simulink model "grid_side_VOC_SteadyState3"  (R2013a)
settings: Solver=ode45  SolverMode=SingleTasking  StartTime=0.0  StopTime=30  FixedStep=0.00001  RelTol=1e-3
values from neighbouring files (symbols this model uses):
  Cdc = 1/(Omega_b*XCdc)    (= 0.0427146921878)    [grid_side_VOC_Constants.m]
  F0 = 1    [grid_side_VOC_Constants.m]
  Fb = 60    [grid_side_VOC_Constants.m]
  Fs = 2040    [grid_side_VOC_Constants.m]
  Fsampling = 10e3    (= 10000)    [grid_side_VOC_Constants.m]
  Grid_Angle_init = pi    (= 3.14159265359)    [grid_side_VOC_Constants.m]
  Ibase = (Pb/3)/(690/(3^0.5))    (= 1924.5008973)    [grid_side_VOC_Constants.m]
  iq_ref_pu = 0    [grid_side_VOC_Constants.m]
  Ki = 2    [grid_side_VOC_Constants.m]
  Kp = 1    [grid_side_VOC_Constants.m]
  Lgrid = 0.1098e-3    (= 0.0001098)    [grid_side_VOC_Constants.m]
  Rdc_series = 0.1*Zb    (= 0.0207)    [grid_side_VOC_Constants.m]
  Vbase = Vp/(2^.5)    (= 398.371685741)    [grid_side_VOC_Constants.m]
  Vdc_ref = 3.062    [grid_side_VOC_Constants.m]
  Vp = (690*(2^0.5))/(3^0.5)    (= 563.38264084)    [grid_side_VOC_Constants.m]
  XLgrid_pu = XLgrid/Zb    (= 0.2)    [grid_side_VOC_Constants.m]
libraries: powerlib x21, powerlib_extras x3, simulink x3, simulink_extras x2
settings Model: Creator=lang  LastModifiedBy=Sony
settings DataIOCC: SignalLoggingSaveFormat=ModelDataLogs
settings OptimizationCC: BlockReduction=off  BooleanDataType=off  InlineParams=on
settings DebuggingCC: SaveWithParameterizedLinksMsg=none  SignalResolutionControl=TryResolveAllWithWarning  SolverPrmCheckMsg=none  MultiTaskDSMMsg=warning  MultiTaskCondExecSysMsg=none  StrictBusMsg=None
settings HardwareCC: TargetUnknown=on
settings RTWCC: IncludeERTFirstTime=on

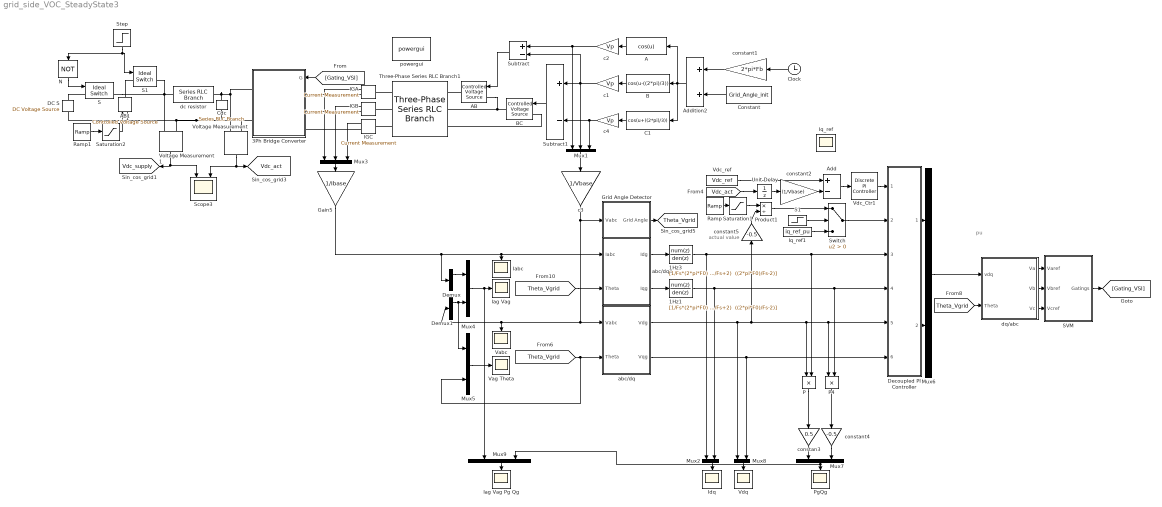
== system grid_side_VOC_SteadyState3 ==
  note: actual value
  note: pu
  " S1" : powerlib/Power Electronics/Ideal Switch  Ron=0  Lon=0  IC=0  Rs=inf  Cs=inf  Measurements=on
  1Hz1 : DiscreteTransferFcn  Numerator=[1/Fs*(2*pi*F0) 1/Fs*(2*pi*F0) ]  Denominator="[((2*pi*F0)/Fs+2)  ((2*pi*F0)/Fs-2)]"  SampleTime=1/Fs
  1Hz3 : DiscreteTransferFcn  Numerator=[1/Fs*(2*pi*F0) 1/Fs*(2*pi*F0) ]  Denominator="[((2*pi*F0)/Fs+2)  ((2*pi*F0)/Fs-2)]"  InitialStates=-250  SampleTime=1/Fs
  3Ph Bridge Converter : Subsystem
  A : Fcn  Expr=cos(u)
  AB : powerlib/Electrical Sources/Controlled Voltage Source  Initialize=off  Source_Type=AC  Amplitude=0  Phase=0  Frequency=0  Measurements=None
  AB1 : powerlib/Electrical Sources/Controlled Voltage Source  Initialize=off  Source_Type=AC  Amplitude=0  Phase=0  Frequency=0  Measurements=None
  Add : Sum  Inputs=+-
  Addition2 : Sum
  B : Fcn  Expr=cos(u-((2*pi)/3))
  BC : powerlib/Electrical Sources/Controlled Voltage Source  Initialize=off  Source_Type=AC  Amplitude=0  Phase=0  Frequency=0  Measurements=None
  C1 : Fcn  Expr=cos(u+((2*pi)/3))
  Cdc : powerlib/Elements/Series RLC Branch  LConnTagsString=__new0  RConnTagsString=__new0  BranchType=C  Resistance=1e-6  Inductance=1e-6  SetiL0=off  InitialCurrent=0  Capacitance=Cdc  Setx0=on  InitialVoltage=Vdc_capacitor_initial  Measurements=None
  Clock : Clock
  Constant : Constant  Value=Grid_Angle_init
  DC S : powerlib/Electrical Sources/DC Voltage Source  Amplitude=1259  Measurements=None
  Decoupled PI Controller : Subsystem
  Demux : Demux  Outputs=3
  Demux1 : Demux  Outputs=3
  Gain5 : Gain  Gain=1/Ibase
  Grid Angle Detector : Subsystem
  IGA : powerlib/Measurements/Current Measurement  PhasorSimulation=off  OutputType=Complex  PSBequivalent=0
  IGB : powerlib/Measurements/Current Measurement  PhasorSimulation=off  OutputType=Complex  PSBequivalent=0
  IGC : powerlib/Measurements/Current Measurement  PhasorSimulation=off  OutputType=Complex  PSBequivalent=0
  Iabc : Scope
      settings: YMin=-2.75  YMax=2.5  SaveName=ScopeData13
  Iag Vag : Scope
      settings: YMin=-1.5  YMax=2  SaveName=ScopeData3
  Iag Vag Pg Qg : Scope
      settings: YMin=-2.25  YMax=2.5  SaveName=ScopeData11
  Idq : Scope
      settings: YMin=-2  YMax=2.25
  Iq_ref : Scope
      settings: YMin=-0.475  YMax=0  SaveName=ScopeData10
  Iq_ref1 : Constant  Value=iq_ref_pu
  Mux1 : Mux  Inputs=3
  Mux{2,4..9} (7 alike) : Mux  Inputs=2
  Mux3 : Mux  Inputs=3
  N : Logic  Operator=NOT  Inputs=1  AllPortsSameDT=off  OutDataTypeStr=boolean
  P : Product
  P4 : Product
  PgQg : Scope
      settings: YMin=-0.67  YMax=-0.47  SaveName=ScopeData7
  Product1 : Product  Inputs=*/
  Ramp : simulink/Sources/Ramp  slope=-10  start=0.15  X0=0
  Ramp1 : simulink/Sources/Ramp  slope=-4000  start=0.05  X0=1259
  S : powerlib/Power Electronics/Ideal Switch  Ron=0  Lon=0  IC=0  Rs=inf  Cs=inf  Measurements=on
  S1 : Step  Time=0.150  SampleTime=0
  SVM : Subsystem
  Saturation1 : Saturate  SampleTime=1/Fsampling
  Saturation2 : Saturate  UpperLimit=1300  LowerLimit=1252  SampleTime=1/Fsampling
  Scope3 : Scope  NumInputPorts=2
      settings: YMin=1100~1025  YMax=1100~1400
  Step : Step  Time=0.050  SampleTime=0
  Subtract : Sum  Inputs=+-
  Subtract1 : Sum  Inputs=+-
  Switch : Switch  Criteria=u2 > Threshold
  Three-Phase Series RLC Branch1 : powerlib/Elements/Three-Phase Series RLC Branch  LConnTagsString=A|B|C  RConnTagsString=A|B|C  BranchType=L  Resistance=1e-6  Inductance=Lgrid  Capacitance=1e-6  Measurements=Branch currents
  Unit Delay : UnitDelay  InitialCondition=1220  SampleTime=1/Fsampling
  Vabc : Scope
      settings: YMin=-1.5  YMax=1.5  SaveName=ScopeData8
  Vag Theta : Scope
      settings: YMin=-1.5  YMax=6.5  SaveName=ScopeData4
  Vdc_Ctr1 : powerlib_extras/Discrete  Control Blocks/Discrete PI Controller  Kp=Kp  Ki=Ki  Par_Limits=[1e6 -1e6]  Init=0  Ts=50e-6
  Vdc_ref : Constant  Value=Vdc_ref
  Vdq : Scope
      settings: YMin=0  YMax=1.5  SaveName=ScopeData9
  Voltage Measurement : powerlib/Measurements/Voltage Measurement  PhasorSimulation=off  OutputType=Complex  PSBequivalent=0
  Voltage Measurement1 : powerlib/Measurements/Voltage Measurement  PhasorSimulation=off  OutputType=Complex  PSBequivalent=0
  abc/dq : Subsystem
  abc/dq1 : Subsystem
  c1 : Gain  Gain=Vp
  c2 : Gain  Gain=Vp
  c3 : Gain  Gain=1/Vbase
  c4 : Gain  Gain=Vp
  constan3 : Gain  Gain=0.5
  constant1 : Gain  Gain=2*pi*Fb
  constant2 : Gain  Gain=(1/Vbase)
  constant4 : Gain  Gain=-0.5
  constant5 : Gain  Gain=-0.5
  dc resistor : powerlib/Elements/Series RLC Branch  LConnTagsString=__new0  RConnTagsString=__new0  BranchType=R  Resistance=Rdc_series  Inductance=1e-3  SetiL0=off  InitialCurrent=0  Capacitance=1e-6  Setx0=off  InitialVoltage=0  Measurements=None
  dq/abc : Subsystem
  powergui : powerlib/powergui  Priority=1  SimulationMode=Continuous  SolverType=Tustin  SampleTime=50e-6  frequency=60  SPID=on  DisableSnubberDevices=off  DisableRonSwitches=off  DisableVfSwitches=off  SwTol=0  Interpol=off  DisplayEquations=off  frequencyindice=0  Pbase=100e6  ErrMax=1e-4  Iterations=50  UnitsV=kV  UnitsW=MW  FunctionMessages=off  echomessages=off  HookPort=off  EnableUseOfTLC=off  x0status=blocks  RestoreLinks=warning  ResistiveCurrentMeasurement=off  Frange=[0:2:500]  Ylog=off  Xlog=on  ShowGrid=off  save=off  variable=ZData  ZoomFFT=off  StartTime=0.0  cycles=1  DisplayStyle=1  fundamental=60  FreqAxis=off  MaxFrequency=1000  frequencyindicesteady=1  RmsSteady=1  display=off  Ts=0  methode=off
  tag scope: Theta_Vgrid=global, Vdc_act=global, Vdc_supply=global
  wires:
  Voltage Measurement/1 -> [Vdc_act], Scope3/2
  Voltage Measurement1/1 -> Scope3/1, [Vdc_supply]
  [Gating_VSI] -> 3Ph Bridge Converter/1(G)
  Step/1 -> " S1"/1, N/1
  N/1 -> S/1
  B/1 -> c1/1
  C1/1 -> c4/1
  Addition2/1 -> C1/1, A/1, B/1
  c1/1 -> Subtract1/1, Mux1/2, Subtract/2
  c4/1 -> Subtract1/2, Mux1/3
  Clock/1 -> constant1/1
  constant1/1 -> Addition2/1
  Constant/1 -> Addition2/2
  IGA/1 -> Mux3/1
  IGB/1 -> Mux3/2
  IGC/1 -> Mux3/3
  Mux3/1 -> Gain5/1
  A/1 -> c2/1
  [Vdc_act] -> Unit Delay/1
  constant2/1 -> Add/2
  Add/1 -> Vdc_Ctr1/1
  Vdc_ref/1 -> Add/1
  Unit Delay/1 -> constant2/1
  Vdc_Ctr1/1 -> Decoupled PI Controller/1(Id_ref)
  Switch/1 -> Decoupled PI Controller/2(Iq_ref)
  Iq_ref1/1 -> Switch/3
  Ramp/1 -> Saturation1/1
  S1/1 -> Switch/2
  Saturation1/1 -> Product1/1
  constant5/1 -> Product1/2
  Product1/1 -> Switch/1
  [Theta_Vgrid] -> dq/abc/2(Theta)
  Decoupled PI Controller/2(vq_ref) -> Mux6/2
  Decoupled PI Controller/1(vd_ref) -> Mux6/1
  Mux6/1 -> dq/abc/1(vdq)
  abc/dq/2(Vqg) -> Mux8/2, Decoupled PI Controller/6(Vq_Grid)
  1Hz1/1 -> Mux2/2, Decoupled PI Controller/4(Iq_VSI), P4/2
  Grid Angle Detector/1(Grid Angle) -> [Theta_Vgrid]
  [Theta_Vgrid] -> Mux5/2, abc/dq/2(Theta)
  dq/abc/1(Va) -> SVM/1(Varef)
  dq/abc/2(Vb) -> SVM/2(Vbref)
  dq/abc/3(Vc) -> SVM/3(Vcref)
  SVM/1(Gatings) -> [Gating_VSI]
  abc/dq/1(Vdg) -> Mux8/1, P/1, Decoupled PI Controller/5(Vd_Grid), P4/1, constant5/1
  c2/1 -> Subtract/1, Mux1/1
  c3/1 -> Grid Angle Detector/1(Vabc), Demux1/1, Vabc/1, abc/dq/1(Vabc)
  Mux2/1 -> Idq/1
  Demux/1 -> Mux4/1
  Gain5/1 -> abc/dq1/1(Iabc), Iabc/1, Demux/1
  Mux5/1 -> Vag Theta/1
  Demux1/1 -> Mux5/1, Mux4/2
  [Theta_Vgrid] -> abc/dq1/2(Theta)
  P/1 -> constan3/1
  P4/1 -> constant4/1
  constan3/1 -> Mux7/1
  constant4/1 -> Mux7/2
  Mux8/1 -> Vdq/1
  Mux4/1 -> Mux9/1, Iag Vag/1
  Mux9/1 -> Iag Vag Pg Qg/1
  Mux7/1 -> Mux9/2, PgQg/1
  abc/dq1/1(Idg) -> 1Hz3/1
  abc/dq1/2(Iqg) -> 1Hz1/1
  1Hz3/1 -> Mux2/1, Decoupled PI Controller/3(Id_VSI), P/2
  Ramp1/1 -> Saturation2/1
  Saturation2/1 -> AB1/1
  Subtract/1 -> AB/1
  Subtract1/1 -> BC/1
  Mux1/1 -> c3/1
  connections:
  Cdc/RConn1 -- dc resistor/RConn1 -- 3Ph Bridge Converter/RConn1 -- Voltage Measurement/LConn1
  3Ph Bridge Converter/RConn2 -- Voltage Measurement/LConn2 -- Cdc/LConn1 -- DC S/LConn1 -- AB1/LConn1 -- Voltage Measurement1/LConn2
  dc resistor/LConn1 -- " S1"/RConn1 -- Voltage Measurement1/LConn1 -- S/RConn1
  IGC/RConn1 -- 3Ph Bridge Converter/LConn3
  S/LConn1 -- DC S/RConn1
  " S1"/LConn1 -- AB1/RConn1
  BC/RConn1 -- AB/LConn1 -- Three-Phase Series RLC Branch1/LConn2
  Three-Phase Series RLC Branch1/RConn2 -- IGB/LConn1
  Three-Phase Series RLC Branch1/RConn3 -- IGC/LConn1
  BC/LConn1 -- Three-Phase Series RLC Branch1/LConn3
  AB/RConn1 -- Three-Phase Series RLC Branch1/LConn1
  3Ph Bridge Converter/LConn2 -- IGB/RConn1
  3Ph Bridge Converter/LConn1 -- IGA/RConn1
  Three-Phase Series RLC Branch1/RConn1 -- IGA/LConn1

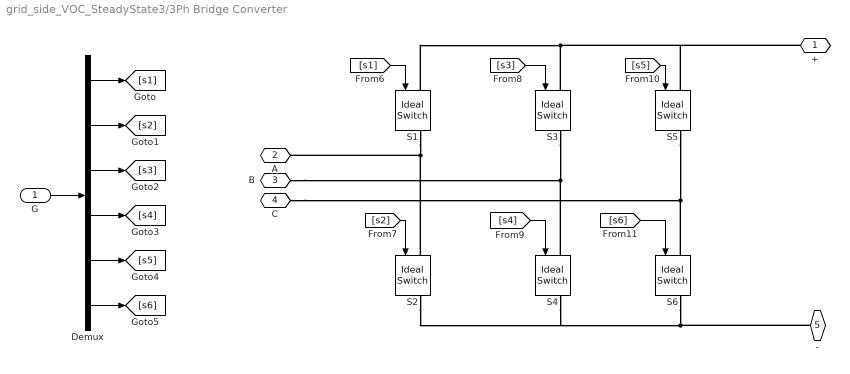
== system grid_side_VOC_SteadyState3/3Ph Bridge Converter ==
  G : Inport
   S{1..6} (6 alike) : powerlib/Power Electronics/Ideal Switch  Ron=0  Lon=0  IC=0  Rs=inf  Cs=inf  Measurements=on
  Demux : Demux  Outputs=6
  + : PMIOPort  Port=1  Side=Right
  A : PMIOPort  Port=2  Side=Left
  B : PMIOPort  Port=3  Side=Left
  C : PMIOPort  Port=4  Side=Left
  - : PMIOPort  Port=5  Side=Right
  wires:
  [s1] -> " S1"/1
  [s5] -> " S5"/1
  Demux/1 -> [s1]
  Demux/2 -> [s2]
  Demux/3 -> [s3]
  Demux/4 -> [s4]
  Demux/5 -> [s5]
  Demux/6 -> [s6]
  G/1 -> Demux/1
  [s2] -> " S2"/1
  [s3] -> " S3"/1
  [s4] -> " S4"/1
  [s6] -> " S6"/1
  connections:
  +/RConn1 -- " S5"/LConn1 -- " S3"/LConn1 -- " S1"/LConn1
  -/RConn1 -- " S2"/RConn1 -- " S4"/RConn1 -- " S6"/RConn1
  " S1"/RConn1 -- " S2"/LConn1 -- A/RConn1
  B/RConn1 -- " S4"/LConn1 -- " S3"/RConn1
  C/RConn1 -- " S6"/LConn1 -- " S5"/RConn1

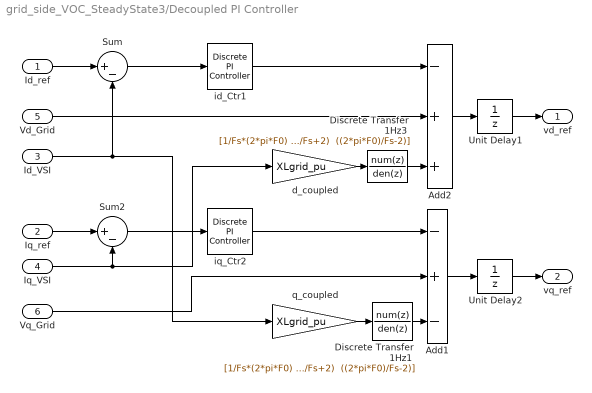
== system grid_side_VOC_SteadyState3/Decoupled PI Controller ==
  Id_ref : Inport
  Iq_ref : Inport  Port=2
  Id_VSI : Inport  Port=3
  Iq_VSI : Inport  Port=4
  Vd_Grid : Inport  Port=5
  Vq_Grid : Inport  Port=6
  Add1 : Sum  Inputs=-+-
  Add2 : Sum  Inputs=-++
  Discrete Transfer 1Hz1 : DiscreteTransferFcn  Numerator=[1/Fs*(2*pi*F0) 1/Fs*(2*pi*F0) ]  Denominator="[((2*pi*F0)/Fs+2)  ((2*pi*F0)/Fs-2)]"  SampleTime=1/Fs
  Discrete Transfer 1Hz3 : DiscreteTransferFcn  Numerator=[1/Fs*(2*pi*F0) 1/Fs*(2*pi*F0) ]  Denominator="[((2*pi*F0)/Fs+2)  ((2*pi*F0)/Fs-2)]"  SampleTime=1/Fs
  Sum : Sum  Inputs=|+-
  Sum2 : Sum  Inputs=|+-
  Unit Delay1 : UnitDelay  SampleTime=1/Fsampling
  Unit Delay2 : UnitDelay  SampleTime=1/Fsampling
  d_coupled : Gain  Gain=XLgrid_pu
  id_Ctr1 : powerlib_extras/Discrete  Control Blocks/Discrete PI Controller  Kp=Kp  Ki=Ki  Par_Limits=[1e6 -1e6]  Init=0  Ts=50e-6
  iq_Ctr2 : powerlib_extras/Discrete  Control Blocks/Discrete PI Controller  Kp=Kp  Ki=Ki  Par_Limits=[1e6 -1e6]  Init=0  Ts=50e-6
  q_coupled : Gain  Gain=XLgrid_pu
  vd_ref : Outport
  vq_ref : Outport  Port=2
  wires:
  id_Ctr1/1 -> Add2/1
  Iq_VSI/1 -> d_coupled/1, Sum2/2
  Sum/1 -> id_Ctr1/1
  iq_Ctr2/1 -> Add1/1
  Vq_Grid/1 -> Add1/2
  Vd_Grid/1 -> Add2/2
  Sum2/1 -> iq_Ctr2/1
  Id_ref/1 -> Sum/1
  Add2/1 -> Unit Delay1/1
  Iq_ref/1 -> Sum2/1
  Add1/1 -> Unit Delay2/1
  d_coupled/1 -> Discrete Transfer 1Hz3/1
  Discrete Transfer 1Hz1/1 -> Add1/3
  Unit Delay2/1 -> vq_ref/1
  Unit Delay1/1 -> vd_ref/1
  Discrete Transfer 1Hz3/1 -> Add2/3
  q_coupled/1 -> Discrete Transfer 1Hz1/1
  Id_VSI/1 -> Sum/2, q_coupled/1

== system grid_side_VOC_SteadyState3/Grid Angle Detector ==
  Vabc : Inport
  Add : Sum
  Beta1 : Fcn  Expr=(1/(3^.5))*(u(1)+2*u(2))
  Cartesian to Polar1 : simulink_extras/Transformations/Cartesian to Polar
  Constant : Constant  Value=2*pi
  Math Function : Math  Operator=rem  SaturateOnIntegerOverflow=on
  Unit Delay3 : UnitDelay  InitialCondition=Grid_Angle_init  SampleTime=1/Fsampling
  alpha1 : Fcn  Expr=u(1)
  Grid Angle : Outport
  wires:
  Beta1/1 -> Cartesian to Polar1/2
  Vabc/1 -> alpha1/1, Beta1/1
  Unit Delay3/1 -> Grid Angle/1
  alpha1/1 -> Cartesian to Polar1/1
  Cartesian to Polar1/2 -> Add/1
  Constant/1 -> Math Function/2, Add/2
  Add/1 -> Math Function/1
  Math Function/1 -> Unit Delay3/1

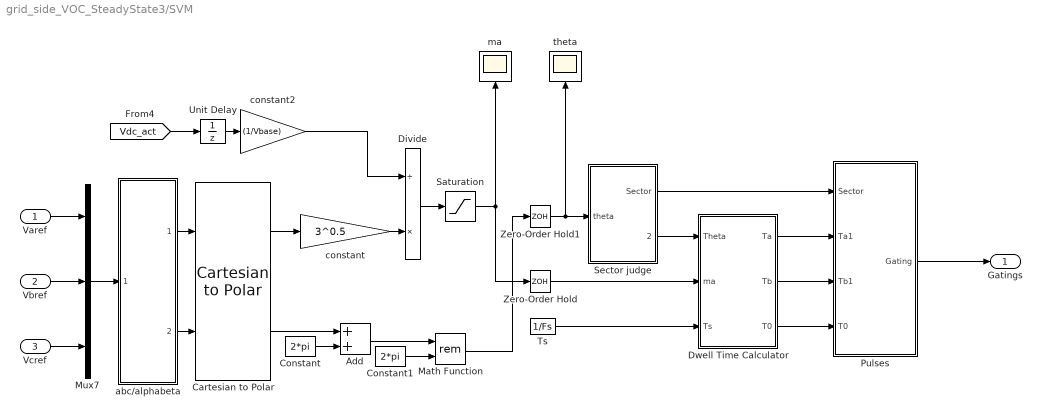
== system grid_side_VOC_SteadyState3/SVM ==
  Varef : Inport
  Vbref : Inport  Port=2
  Vcref : Inport  Port=3
  Add : Sum
  Cartesian to Polar : simulink_extras/Transformations/Cartesian to Polar
  Constant : Constant  Value=2*pi
  Constant1 : Constant  Value=2*pi
  Divide : Product  Inputs=/*
  Dwell Time Calculator : Subsystem
  Math Function : Math  Operator=rem  SaturateOnIntegerOverflow=on
  Mux7 : Mux  Inputs=3
  Pulses : Subsystem
  Saturation : Saturate  UpperLimit=1  LowerLimit=0  SampleTime=1/Fsampling
  Sector judge : Subsystem
  Ts : Constant  Value=1/Fs
  Unit Delay : UnitDelay  InitialCondition=1220  SampleTime=1/Fsampling
  Zero-Order Hold : ZeroOrderHold  SampleTime=1/(2*Fs)
  Zero-Order Hold1 : ZeroOrderHold  SampleTime=1/(2*Fs)
  abc/alphabeta : Subsystem
  constant : Gain  Gain=3^0.5
  constant2 : Gain  Gain=(1/Vbase)
  ma : Scope
      settings: SaveName=ScopeData5
  theta : Scope
      settings: YMin=-3.5  YMax=3.5  SaveName=ScopeData6
  Gatings : Outport
  wires:
  Dwell Time Calculator/3(T0) -> Pulses/4(T0)
  constant/1 -> Divide/2
  Pulses/1(Gating) -> Gatings/1
  Cartesian to Polar/1 -> constant/1
  Divide/1 -> Saturation/1
  Ts/1 -> Dwell Time Calculator/3(Ts)
  Varef/1 -> Mux7/1
  Dwell Time Calculator/1(Ta) -> Pulses/2(Ta1)
  Dwell Time Calculator/2(Tb) -> Pulses/3(Tb1)
  Sector judge/2(Cal_theta) -> Dwell Time Calculator/1(Theta)
  Saturation/1 -> Zero-Order Hold/1, ma/1
  Zero-Order Hold/1 -> Dwell Time Calculator/2(ma)
  constant2/1 -> Divide/1
  Zero-Order Hold1/1 -> Sector judge/1(theta), theta/1
  Sector judge/1(Sector) -> Pulses/1(Sector)
  abc/alphabeta/1(Valpha) -> Cartesian to Polar/1
  Mux7/1 -> abc/alphabeta/1(Vabc)
  Vbref/1 -> Mux7/2
  abc/alphabeta/2(Vbeta) -> Cartesian to Polar/2
  Vcref/1 -> Mux7/3
  Cartesian to Polar/2 -> Add/1
  Math Function/1 -> Zero-Order Hold1/1
  Constant/1 -> Add/2
  Add/1 -> Math Function/1
  Constant1/1 -> Math Function/2
  [Vdc_act] -> Unit Delay/1
  Unit Delay/1 -> constant2/1

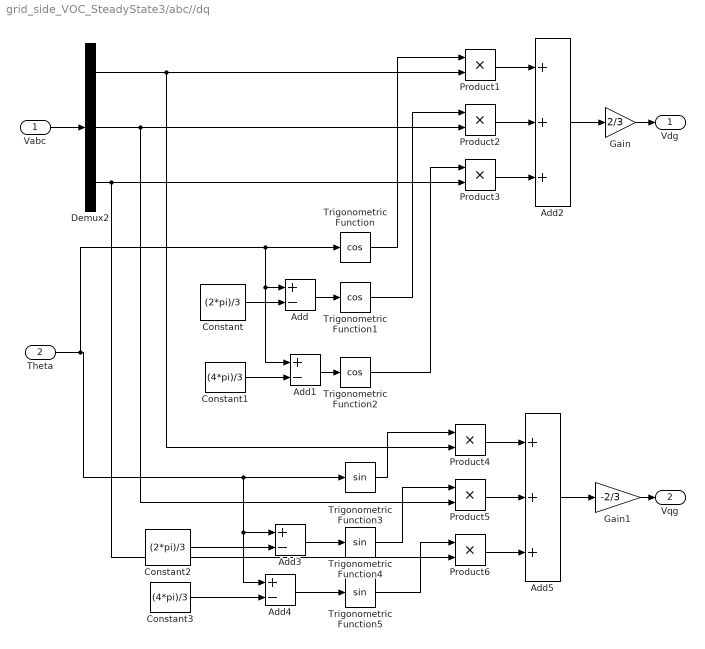
== system grid_side_VOC_SteadyState3/abc//dq ==
  Vabc : Inport
  Theta : Inport  Port=2
  Add{,1,3..4} (4 alike) : Sum  Inputs=+-
  Add2 : Sum  Inputs=+++
  Add5 : Sum  Inputs=+++
  Constant : Constant  Value=(2*pi)/3
  Constant1 : Constant  Value=(4*pi)/3
  Constant2 : Constant  Value=(2*pi)/3
  Constant3 : Constant  Value=(4*pi)/3
  Demux2 : Demux  Outputs=3
  Gain : Gain  Gain=2/3
  Gain1 : Gain  Gain=-2/3
  Product{1..6} (6 alike) : Product
  Trigonometric Function : Trigonometry  Operator=cos
  Trigonometric Function1 : Trigonometry  Operator=cos
  Trigonometric Function2 : Trigonometry  Operator=cos
  Trigonometric Function3 : Trigonometry
  Trigonometric Function4 : Trigonometry
  Trigonometric Function5 : Trigonometry
  Vdg : Outport
  Vqg : Outport  Port=2
  wires:
  Trigonometric Function1/1 -> Product2/1
  Constant/1 -> Add/2
  Trigonometric Function/1 -> Product1/1
  Trigonometric Function2/1 -> Product3/1
  Add/1 -> Trigonometric Function1/1
  Constant1/1 -> Add1/2
  Product2/1 -> Add2/2
  Product1/1 -> Add2/1
  Constant2/1 -> Add3/2
  Demux2/1 -> Product4/2, Product1/2
  Product5/1 -> Add5/2
  Constant3/1 -> Add4/2
  Add4/1 -> Trigonometric Function5/1
  Trigonometric Function3/1 -> Product4/1
  Trigonometric Function4/1 -> Product5/1
  Add3/1 -> Trigonometric Function4/1
  Trigonometric Function5/1 -> Product6/1
  Demux2/2 -> Product5/2, Product2/2
  Demux2/3 -> Product6/2, Product3/2
  Product4/1 -> Add5/1
  Add5/1 -> Gain1/1
  Product6/1 -> Add5/3
  Add1/1 -> Trigonometric Function2/1
  Product3/1 -> Add2/3
  Theta/1 -> Trigonometric Function/1, Add1/1, Add/1, Add4/1, Add3/1, Trigonometric Function3/1
  Vabc/1 -> Demux2/1
  Gain/1 -> Vdg/1
  Add2/1 -> Gain/1
  Gain1/1 -> Vqg/1

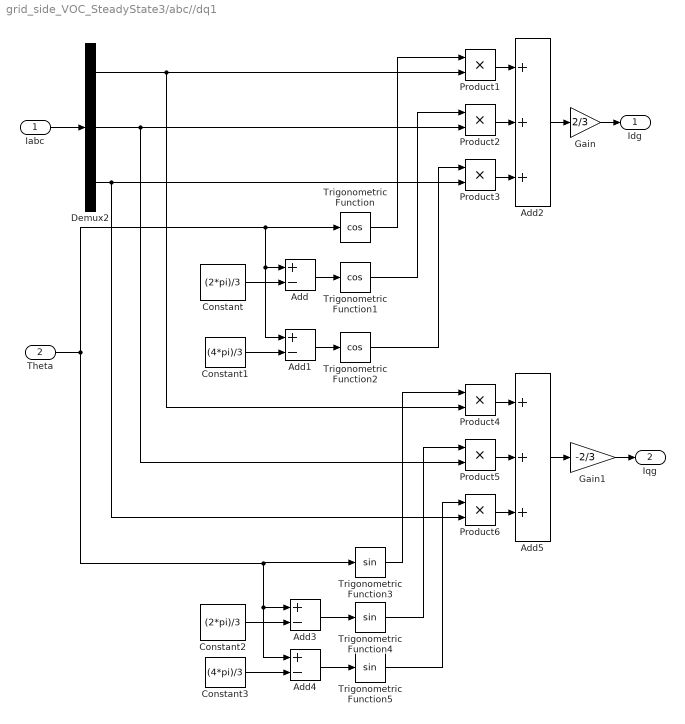
== system grid_side_VOC_SteadyState3/abc//dq1 ==
  Iabc : Inport
  Theta : Inport  Port=2
  Add{,1,3..4} (4 alike) : Sum  Inputs=+-
  Add2 : Sum  Inputs=+++
  Add5 : Sum  Inputs=+++
  Constant : Constant  Value=(2*pi)/3
  Constant1 : Constant  Value=(4*pi)/3
  Constant2 : Constant  Value=(2*pi)/3
  Constant3 : Constant  Value=(4*pi)/3
  Demux2 : Demux  Outputs=3
  Gain : Gain  Gain=2/3
  Gain1 : Gain  Gain=-2/3
  Product{1..6} (6 alike) : Product
  Trigonometric Function : Trigonometry  Operator=cos
  Trigonometric Function1 : Trigonometry  Operator=cos
  Trigonometric Function2 : Trigonometry  Operator=cos
  Trigonometric Function3 : Trigonometry
  Trigonometric Function4 : Trigonometry
  Trigonometric Function5 : Trigonometry
  Idg : Outport
  Iqg : Outport  Port=2
  wires:
  Trigonometric Function1/1 -> Product2/1
  Constant/1 -> Add/2
  Trigonometric Function/1 -> Product1/1
  Trigonometric Function2/1 -> Product3/1
  Add/1 -> Trigonometric Function1/1
  Constant1/1 -> Add1/2
  Product2/1 -> Add2/2
  Product1/1 -> Add2/1
  Constant2/1 -> Add3/2
  Demux2/1 -> Product4/2, Product1/2
  Product5/1 -> Add5/2
  Constant3/1 -> Add4/2
  Add4/1 -> Trigonometric Function5/1
  Trigonometric Function3/1 -> Product4/1
  Trigonometric Function4/1 -> Product5/1
  Add3/1 -> Trigonometric Function4/1
  Trigonometric Function5/1 -> Product6/1
  Demux2/2 -> Product5/2, Product2/2
  Demux2/3 -> Product6/2, Product3/2
  Product4/1 -> Add5/1
  Add5/1 -> Gain1/1
  Product6/1 -> Add5/3
  Add1/1 -> Trigonometric Function2/1
  Product3/1 -> Add2/3
  Theta/1 -> Trigonometric Function/1, Add1/1, Add/1, Add4/1, Add3/1, Trigonometric Function3/1
  Gain1/1 -> Iqg/1
  Iabc/1 -> Demux2/1
  Gain/1 -> Idg/1
  Add2/1 -> Gain/1

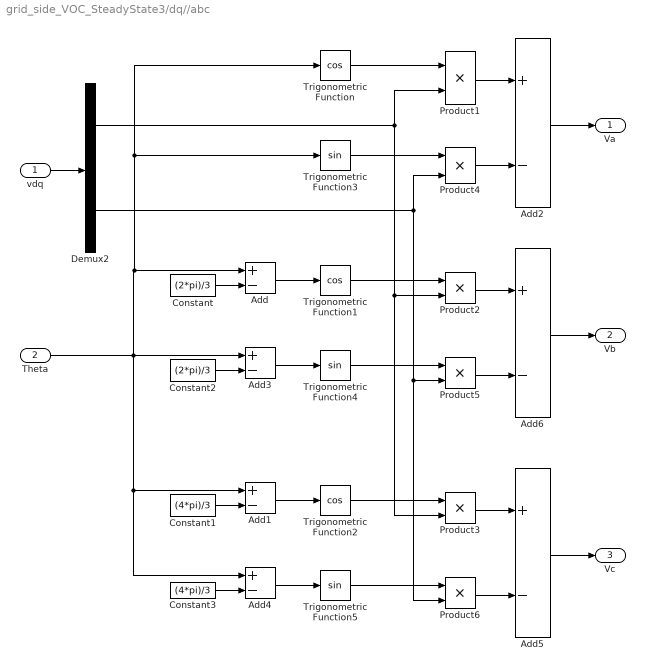
== system grid_side_VOC_SteadyState3/dq//abc ==
  vdq : Inport
  Theta : Inport  Port=2
  Add{,1..6} (7 alike) : Sum  Inputs=+-
  Constant : Constant  Value=(2*pi)/3
  Constant1 : Constant  Value=(4*pi)/3
  Constant2 : Constant  Value=(2*pi)/3
  Constant3 : Constant  Value=(4*pi)/3
  Demux2 : Demux  Outputs=2
  Product{1..6} (6 alike) : Product
  Trigonometric Function : Trigonometry  Operator=cos
  Trigonometric Function1 : Trigonometry  Operator=cos
  Trigonometric Function2 : Trigonometry  Operator=cos
  Trigonometric Function3 : Trigonometry
  Trigonometric Function4 : Trigonometry
  Trigonometric Function5 : Trigonometry
  Va : Outport
  Vb : Outport  Port=2
  Vc : Outport  Port=3
  wires:
  Trigonometric Function1/1 -> Product2/1
  Constant/1 -> Add/2
  Trigonometric Function/1 -> Product1/1
  Add/1 -> Trigonometric Function1/1
  Product1/1 -> Add2/1
  Constant2/1 -> Add3/2
  Demux2/1 -> Product1/2, Product2/2, Product3/2
  Trigonometric Function3/1 -> Product4/1
  Trigonometric Function4/1 -> Product5/1
  Add3/1 -> Trigonometric Function4/1
  vdq/1 -> Demux2/1
  Add2/1 -> Va/1
  Product4/1 -> Add2/2
  Demux2/2 -> Product4/2, Product6/2, Product5/2
  Product2/1 -> Add6/1
  Add6/1 -> Vb/1
  Product5/1 -> Add6/2
  Trigonometric Function2/1 -> Product3/1
  Constant1/1 -> Add1/2
  Add1/1 -> Trigonometric Function2/1
  Constant3/1 -> Add4/2
  Trigonometric Function5/1 -> Product6/1
  Add4/1 -> Trigonometric Function5/1
  Theta/1 -> Trigonometric Function/1, Trigonometric Function3/1, Add/1, Add4/1, Add1/1, Add3/1
  Product3/1 -> Add5/1
  Add5/1 -> Vc/1
  Product6/1 -> Add5/2

== system grid_side_VOC_SteadyState3/SVM/Dwell Time Calculator ==
  Theta : Inport
  ma : Inport  Port=2
  Ts : Inport  Port=3
  Add : Sum  Inputs=--+
  Compare To Zero : simulink/Logic and Bit Operations/Compare To Zero  relop=>=  OutDataTypeStr=boolean
  Data Type Conversion : DataTypeConversion  OutDataTypeStr=double
  Mux : Mux  Inputs=3
  Product : Product  RndMeth=Zero
  Scope : Scope  NumInputPorts=3
      settings: YMin=-5~-5~-5  YMax=5~5~5  SaveName=ScopeData12
  cTa : Fcn  Expr=u(2)*u(3)*sin((pi/3)-u(1))
  cTb : Fcn  Expr=u(2)*u(3)*sin(u(1))
  Ta : Outport
  Tb : Outport  Port=2
  T0 : Outport  Port=3
  wires:
  Product/1 -> Scope/1, T0/1
  Theta/1 -> Mux/1
  ma/1 -> Mux/2
  Ts/1 -> Add/3, Mux/3
  Mux/1 -> cTb/1, cTa/1
  Add/1 -> Product/2, Compare To Zero/1
  Data Type Conversion/1 -> Product/1
  Compare To Zero/1 -> Data Type Conversion/1
  cTa/1 -> Scope/2, Ta/1, Add/1
  cTb/1 -> Scope/3, Tb/1, Add/2

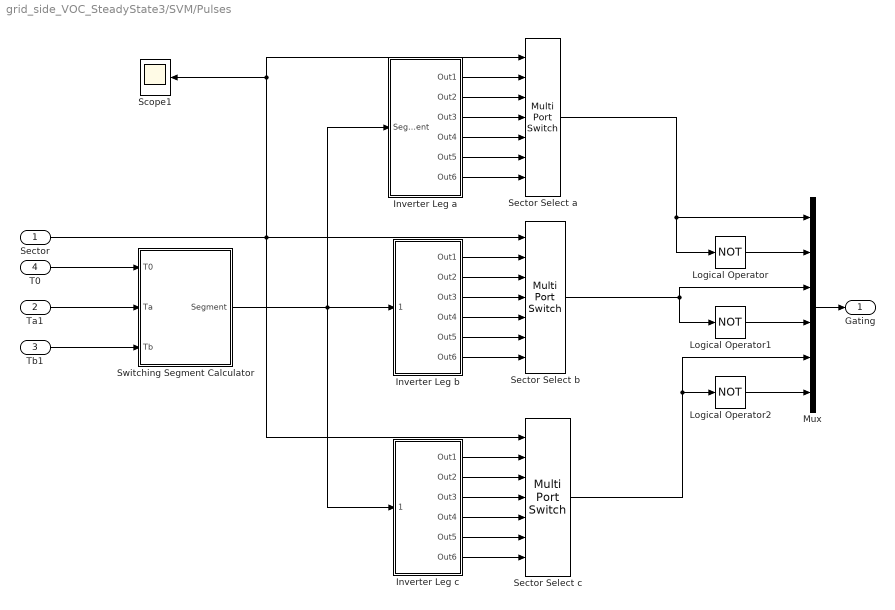
== system grid_side_VOC_SteadyState3/SVM/Pulses ==
  Sector : Inport
  Ta1 : Inport  Port=2
  Tb1 : Inport  Port=3
  T0 : Inport  Port=4
  Inverter Leg a : Subsystem
  Inverter Leg b : Subsystem
  Inverter Leg c : Subsystem
  Logical Operator : Logic  Operator=NOT  AllPortsSameDT=off
  Logical Operator1 : Logic  Operator=NOT  AllPortsSameDT=off
  Logical Operator2 : Logic  Operator=NOT  AllPortsSameDT=off
  Mux : Mux  Inputs=6
  Scope1 : Scope
      settings: SaveName=ScopeData2
  Sector Select a : MultiPortSwitch  Inputs=6
  Sector Select b : MultiPortSwitch  Inputs=6
  Sector Select c : MultiPortSwitch  Inputs=6
  Switching Segment Calculator : Subsystem
  Gating : Outport
  wires:
  Sector/1 -> Sector Select a/1, Scope1/1, Sector Select b/1, Sector Select c/1
  Sector Select a/1 -> Logical Operator/1, Mux/1
  Sector Select b/1 -> Logical Operator1/1, Mux/3
  Sector Select c/1 -> Logical Operator2/1, Mux/5
  Mux/1 -> Gating/1
  Logical Operator/1 -> Mux/2
  Logical Operator1/1 -> Mux/4
  Logical Operator2/1 -> Mux/6
  Switching Segment Calculator/1(Segment) -> Inverter Leg c/1(Segment), Inverter Leg a/1(Segment), Inverter Leg b/1(Segment)
  T0/1 -> Switching Segment Calculator/1(T0)
  Ta1/1 -> Switching Segment Calculator/2(Ta)
  Tb1/1 -> Switching Segment Calculator/3(Tb)
  Inverter Leg a/1(Out1) -> Sector Select a/2
  Inverter Leg a/2(Out2) -> Sector Select a/3
  Inverter Leg a/3(Out3) -> Sector Select a/4
  Inverter Leg a/4(Out4) -> Sector Select a/5
  Inverter Leg a/5(Out5) -> Sector Select a/6
  Inverter Leg a/6(Out6) -> Sector Select a/7
  Inverter Leg b/1(Out1) -> Sector Select b/2
  Inverter Leg b/2(Out2) -> Sector Select b/3
  Inverter Leg b/3(Out3) -> Sector Select b/4
  Inverter Leg b/4(Out4) -> Sector Select b/5
  Inverter Leg b/5(Out5) -> Sector Select b/6
  Inverter Leg b/6(Out6) -> Sector Select b/7
  Inverter Leg c/1(Out1) -> Sector Select c/2
  Inverter Leg c/2(Out2) -> Sector Select c/3
  Inverter Leg c/3(Out3) -> Sector Select c/4
  Inverter Leg c/4(Out4) -> Sector Select c/5
  Inverter Leg c/5(Out5) -> Sector Select c/6
  Inverter Leg c/6(Out6) -> Sector Select c/7

== system grid_side_VOC_SteadyState3/SVM/Sector judge ==
  theta : Inport
  Add : Sum
  Constant : Constant  Value=2*pi
  Constant1 : Constant  OutDataTypeStr=boolean
  Constant2 : Constant  Value=2*pi
  Gain1 : Gain  Gain=3/pi
  Gain2 : Gain  Gain=pi/3
  Math Function1 : Math  Operator=rem  SaturateOnIntegerOverflow=on
  Rounding Function : Rounding
  Sum1 : Sum  Inputs=|++  SaturateOnIntegerOverflow=on
  Sum2 : Sum  Inputs=|-+
  Sector : Outport
  Cal_theta : Outport  Port=2
  wires:
  Gain1/1 -> Rounding Function/1
  Rounding Function/1 -> Gain2/1, Sum1/1
  Sum1/1 -> Sector/1
  Constant1/1 -> Sum1/2
  Gain2/1 -> Sum2/1
  Sum2/1 -> Cal_theta/1
  theta/1 -> Add/1
  Math Function1/1 -> Sum2/2, Gain1/1
  Constant/1 -> Add/2
  Add/1 -> Math Function1/1
  Constant2/1 -> Math Function1/2

== system grid_side_VOC_SteadyState3/SVM/abc//alphabeta ==
  Vabc : Inport
  Beta1 : Fcn  Expr=(1/(3^.5))*(u(1)+2*u(2))
  alpha1 : Fcn  Expr=u(1)
  Valpha : Outport
  Vbeta : Outport  Port=2
  wires:
  Vabc/1 -> Beta1/1, alpha1/1
  alpha1/1 -> Valpha/1
  Beta1/1 -> Vbeta/1

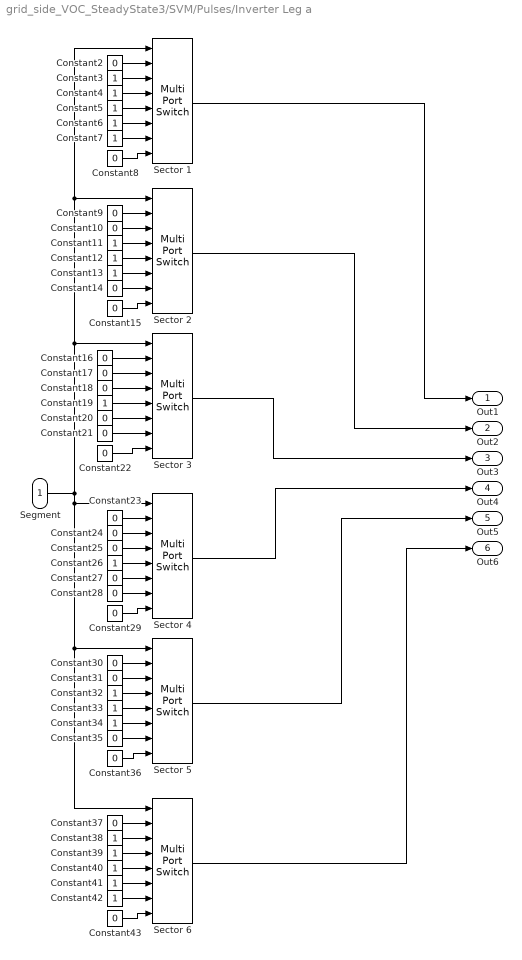
== system grid_side_VOC_SteadyState3/SVM/Pulses/Inverter Leg a ==
  Segment : Inport
  Constant{2,8..10,14..18,20..25,27..31,35..37,43} (24 alike) : Constant  Value=0
  Constant{3..7,11..13,19,26,32..34,38..42} (18 alike) : Constant
  Sector {1..6} (6 alike) : MultiPortSwitch  Inputs=7
  Out1 : Outport
  Out2 : Outport  Port=2
  Out3 : Outport  Port=3
  Out4 : Outport  Port=4
  Out5 : Outport  Port=5
  Out6 : Outport  Port=6
  wires:
  Segment/1 -> Sector 6/1, Sector 5/1, Sector 4/1, Sector 2/1, Sector 1/1, Sector 3/1
  Sector 3/1 -> Out3/1
  Constant2/1 -> Sector 1/2
  Constant7/1 -> Sector 1/7
  Sector 1/1 -> Out1/1
  Constant3/1 -> Sector 1/3
  Constant6/1 -> Sector 1/6
  Constant10/1 -> Sector 2/3
  Sector 6/1 -> Out6/1
  Sector 2/1 -> Out2/1
  Constant5/1 -> Sector 1/5
  Constant9/1 -> Sector 2/2
  Constant4/1 -> Sector 1/4
  Constant8/1 -> Sector 1/8
  Sector 4/1 -> Out4/1
  Sector 5/1 -> Out5/1
  Constant42/1 -> Sector 6/7
  Constant43/1 -> Sector 6/8
  Constant40/1 -> Sector 6/5
  Constant37/1 -> Sector 6/2
  Constant41/1 -> Sector 6/6
  Constant39/1 -> Sector 6/4
  Constant17/1 -> Sector 3/3
  Constant30/1 -> Sector 5/2
  Constant38/1 -> Sector 6/3
  Constant29/1 -> Sector 4/8
  Constant28/1 -> Sector 4/7
  Constant31/1 -> Sector 5/3
  Constant25/1 -> Sector 4/4
  Constant20/1 -> Sector 3/6
  Constant26/1 -> Sector 4/5
  Constant32/1 -> Sector 5/4
  Constant33/1 -> Sector 5/5
  Constant36/1 -> Sector 5/8
  Constant18/1 -> Sector 3/4
  Constant14/1 -> Sector 2/7
  Constant13/1 -> Sector 2/6
  Constant34/1 -> Sector 5/6
  Constant24/1 -> Sector 4/3
  Constant11/1 -> Sector 2/4
  Constant16/1 -> Sector 3/2
  Constant21/1 -> Sector 3/7
  Constant12/1 -> Sector 2/5
  Constant19/1 -> Sector 3/5
  Constant35/1 -> Sector 5/7
  Constant22/1 -> Sector 3/8
  Constant23/1 -> Sector 4/2
  Constant15/1 -> Sector 2/8
  Constant27/1 -> Sector 4/6

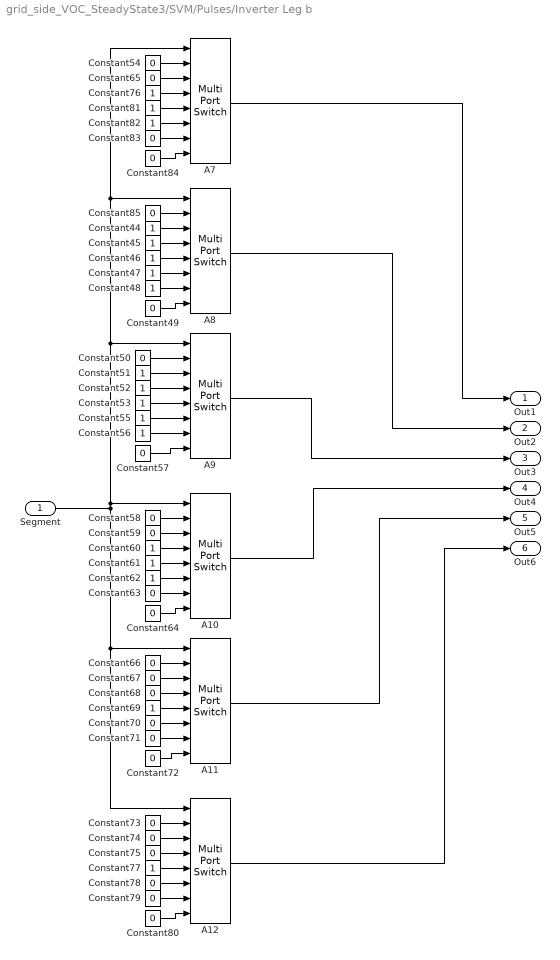
== system grid_side_VOC_SteadyState3/SVM/Pulses/Inverter Leg b ==
  Segment : Inport
  A{7..12} (6 alike) : MultiPortSwitch  Inputs=7
  Constant{44..48,51..53,55..56,60..62,69,76..77,81..82} (18 alike) : Constant
  Constant{49..50,54,57..59,63..68,70..75,78..80,83..85} (24 alike) : Constant  Value=0
  Out1 : Outport
  Out2 : Outport  Port=2
  Out3 : Outport  Port=3
  Out4 : Outport  Port=4
  Out5 : Outport  Port=5
  Out6 : Outport  Port=6
  wires:
  Segment/1 -> A7/1, A8/1, A9/1, A10/1, A12/1, A11/1
  Constant80/1 -> A12/8
  Constant71/1 -> A11/7
  Constant69/1 -> A11/5
  Constant70/1 -> A11/6
  Constant72/1 -> A11/8
  Constant73/1 -> A12/2
  Constant75/1 -> A12/4
  Constant77/1 -> A12/5
  Constant79/1 -> A12/7
  Constant74/1 -> A12/3
  Constant68/1 -> A11/4
  Constant78/1 -> A12/6
  Constant55/1 -> A9/6
  Constant61/1 -> A10/5
  Constant47/1 -> A8/6
  Constant53/1 -> A9/5
  Constant45/1 -> A8/4
  Constant85/1 -> A8/2
  Constant49/1 -> A8/8
  Constant52/1 -> A9/4
  Constant56/1 -> A9/7
  Constant51/1 -> A9/3
  Constant57/1 -> A9/8
  Constant44/1 -> A8/3
  Constant46/1 -> A8/5
  Constant50/1 -> A9/2
  Constant48/1 -> A8/7
  Constant60/1 -> A10/4
  Constant62/1 -> A10/6
  Constant63/1 -> A10/7
  Constant64/1 -> A10/8
  Constant67/1 -> A11/3
  Constant66/1 -> A11/2
  Constant84/1 -> A7/8
  Constant59/1 -> A10/3
  Constant58/1 -> A10/2
  A9/1 -> Out3/1
  A8/1 -> Out2/1
  Constant65/1 -> A7/3
  A12/1 -> Out6/1
  A11/1 -> Out5/1
  A7/1 -> Out1/1
  Constant54/1 -> A7/2
  Constant76/1 -> A7/4
  A10/1 -> Out4/1
  Constant81/1 -> A7/5
  Constant82/1 -> A7/6
  Constant83/1 -> A7/7

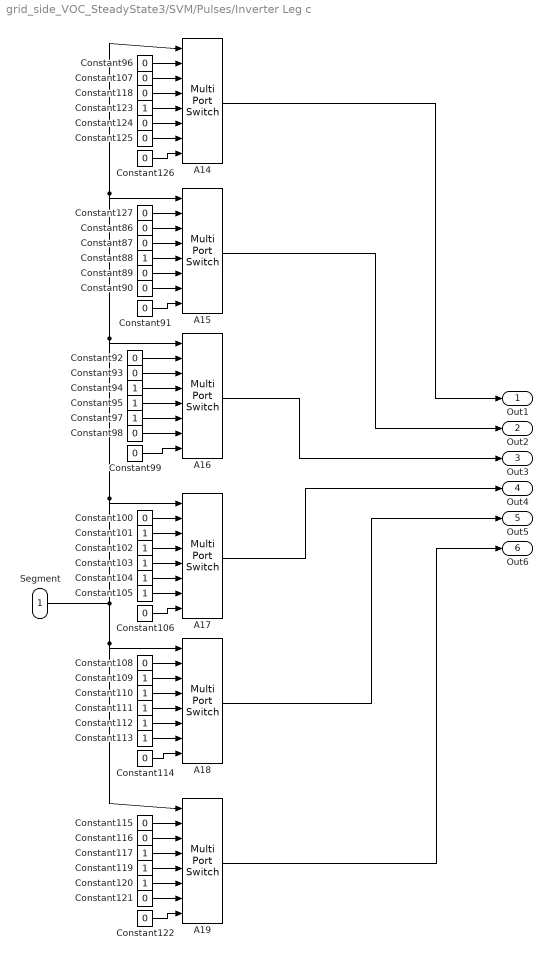
== system grid_side_VOC_SteadyState3/SVM/Pulses/Inverter Leg c ==
  Segment : Inport
  A{14..19} (6 alike) : MultiPortSwitch  Inputs=7
  Constant{86..87,89..93,96,98..100,106..108,114..116,118,121..122,124..127} (24 alike) : Constant  Value=0
  Constant{88,94..95,97,101..105,109..113,117,119..120,123} (18 alike) : Constant
  Out1 : Outport
  Out2 : Outport  Port=2
  Out3 : Outport  Port=3
  Out4 : Outport  Port=4
  Out5 : Outport  Port=5
  Out6 : Outport  Port=6
  wires:
  Constant86/1 -> A15/3
  Constant103/1 -> A17/5
  Constant88/1 -> A15/5
  Constant101/1 -> A17/3
  Constant127/1 -> A15/2
  Constant102/1 -> A17/4
  Constant104/1 -> A17/6
  Constant100/1 -> A17/2
  Constant97/1 -> A16/6
  Constant94/1 -> A16/4
  Constant99/1 -> A16/8
  Constant105/1 -> A17/7
  Constant110/1 -> A18/4
  Constant109/1 -> A18/3
  Constant89/1 -> A15/6
  Constant113/1 -> A18/7
  Constant114/1 -> A18/8
  Constant87/1 -> A15/4
  Constant98/1 -> A16/7
  Constant91/1 -> A15/8
  Constant108/1 -> A18/2
  Constant92/1 -> A16/2
  Constant116/1 -> A19/3
  Constant111/1 -> A18/5
  Constant115/1 -> A19/2
  Constant117/1 -> A19/4
  Constant119/1 -> A19/5
  Constant112/1 -> A18/6
  Constant93/1 -> A16/3
  Constant95/1 -> A16/5
  Constant90/1 -> A15/7
  Constant106/1 -> A17/8
  Constant122/1 -> A19/8
  Constant121/1 -> A19/7
  Constant120/1 -> A19/6
  Segment/1 -> A15/1, A14/1, A16/1, A17/1, A19/1, A18/1
  Constant126/1 -> A14/8
  A16/1 -> Out3/1
  A17/1 -> Out4/1
  Constant96/1 -> A14/2
  Constant118/1 -> A14/4
  A18/1 -> Out5/1
  Constant107/1 -> A14/3
  A19/1 -> Out6/1
  Constant123/1 -> A14/5
  A15/1 -> Out2/1
  Constant124/1 -> A14/6
  A14/1 -> Out1/1
  Constant125/1 -> A14/7

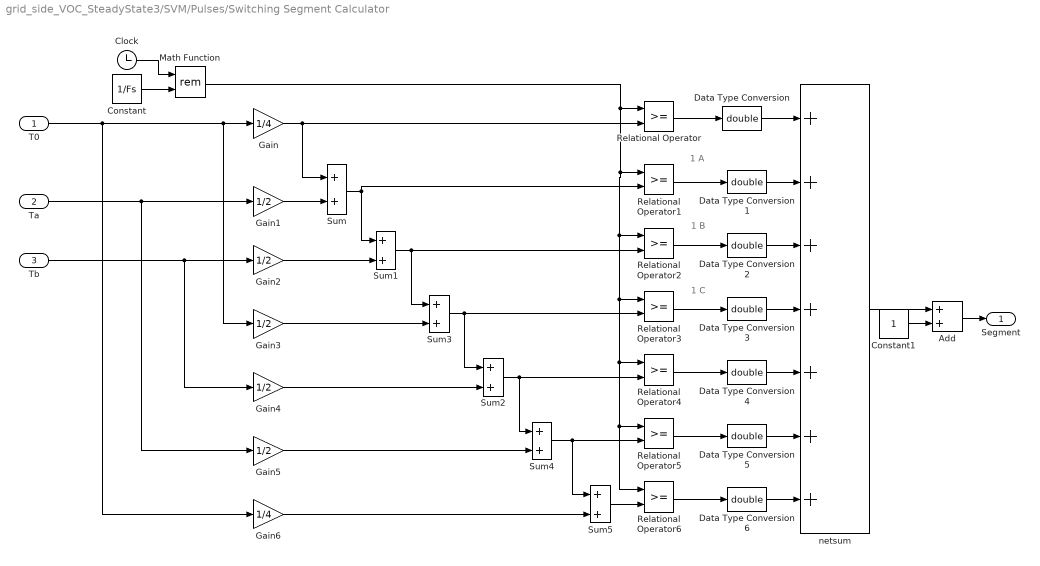
== system grid_side_VOC_SteadyState3/SVM/Pulses/Switching Segment Calculator ==
  note: 1 A
  note: 1 B
  note: 1 C
  T0 : Inport
  Ta : Inport  Port=2
  Tb : Inport  Port=3
  Add : Sum
  Clock : Clock
  Constant : Constant  Value=1/Fs
  Constant1 : Constant
  Data Type Conversion{,1..6} (7 alike) : DataTypeConversion  OutDataTypeStr=double
  Gain : Gain  Gain=1/4
  Gain{1..5} (5 alike) : Gain  Gain=1/2
  Gain6 : Gain  Gain=1/4
  Math Function : Math  Operator=rem  SaturateOnIntegerOverflow=on
  Relational Operator{,1..6} (7 alike) : RelationalOperator  OutDataTypeStr=boolean
  Sum{,1..5} (6 alike) : Sum
  netsum : Sum  Inputs=7  SaturateOnIntegerOverflow=on  InputSameDT=on  OutDataTypeStr=Inherit: Same as first input
  Segment : Outport
  wires:
  Ta/1 -> Gain5/1, Gain1/1
  Gain2/1 -> Sum1/2
  Sum4/1 -> Sum5/1, Relational Operator5/2
  Math Function/1 -> Relational Operator6/1, Relational Operator5/1, Relational Operator4/1, Relational Operator3/1, Relational Operator2/1, Relational Operator1/1, Relational Operator/1
  Gain4/1 -> Sum2/2
  Gain5/1 -> Sum4/2
  Relational Operator/1 -> Data Type Conversion/1
  Relational Operator1/1 -> Data Type Conversion1/1
  Relational Operator2/1 -> Data Type Conversion2/1
  Sum3/1 -> Sum2/1, Relational Operator3/2
  Constant/1 -> Math Function/2
  Relational Operator3/1 -> Data Type Conversion3/1
  Gain3/1 -> Sum3/2
  Sum5/1 -> Relational Operator6/2
  Sum1/1 -> Sum3/1, Relational Operator2/2
  Gain6/1 -> Sum5/2
  Clock/1 -> Math Function/1
  Tb/1 -> Gain4/1, Gain2/1
  Sum/1 -> Sum1/1, Relational Operator1/2
  Gain/1 -> Sum/1, Relational Operator/2
  Gain1/1 -> Sum/2
  Sum2/1 -> Sum4/1, Relational Operator4/2
  Data Type Conversion3/1 -> netsum/4
  netsum/1 -> Add/1
  Data Type Conversion2/1 -> netsum/3
  Constant1/1 -> Add/2
  Data Type Conversion1/1 -> netsum/2
  Relational Operator4/1 -> Data Type Conversion4/1
  Data Type Conversion4/1 -> netsum/5
  Data Type Conversion6/1 -> netsum/7
  Data Type Conversion/1 -> netsum/1
  Relational Operator6/1 -> Data Type Conversion6/1
  Data Type Conversion5/1 -> netsum/6
  Relational Operator5/1 -> Data Type Conversion5/1
  Add/1 -> Segment/1
  T0/1 -> Gain6/1, Gain3/1, Gain/1
